simulink model "Pacemaker_Model"  (R2020a)
settings: Solver=FixedStepAuto  StartTime=0.0  StopTime=inf  FixedStep=1e-3  RelTol=1e-3  EnableMultiTasking=on
undefined symbols (not defined in the file): A0, A1, magnitude, PTB2, PTB3
libraries: etargetslib x7, frdmk64flib x5, dspstat3 x1
settings Model: ExtModeTrigDuration=5  Creator=iceca  LastModifiedBy=iceca
settings OptimizationCC: EnhancedBackFolding=on  PassReuseOutputArgsAs=Individual arguments  ZeroExternalMemoryAtStartup=off  ZeroInternalMemoryAtStartup=off  MaxStackSize=64  OptimizeBlockOrder=speed  DifferentSizesBufferReuse=on  OptimizationCustomize=off  EfficientTunableParamExpr=on
settings DebuggingCC: ParameterTunabilityLossMsg=error
settings HardwareCC: ProdBitPerPointer=32  ProdBitPerSizeT=32  ProdBitPerPtrDiffT=32  ProdLargestAtomicInteger=Long  ProdLargestAtomicFloat=Double  ProdWordSize=32  ProdHWDeviceType=ARM Compatible->ARM Cortex
settings SFSimCC: MATLABDynamicMemAlloc=off
settings RTWCC: SystemTargetFile=ert.tlc  HardwareBoard=NXP FRDM-K64F  TemplateMakefile=ert_default_tmf  Toolchain=GNU Tools for ARM Embedded Processors
settings CodeAppCC: ForceParamTrailComments=on  IgnoreCustomStorageClasses=off  OperatorAnnotations=on  SimulinkDataObjDesc=on  SFDataObjDesc=on  InsertBlockDesc=on

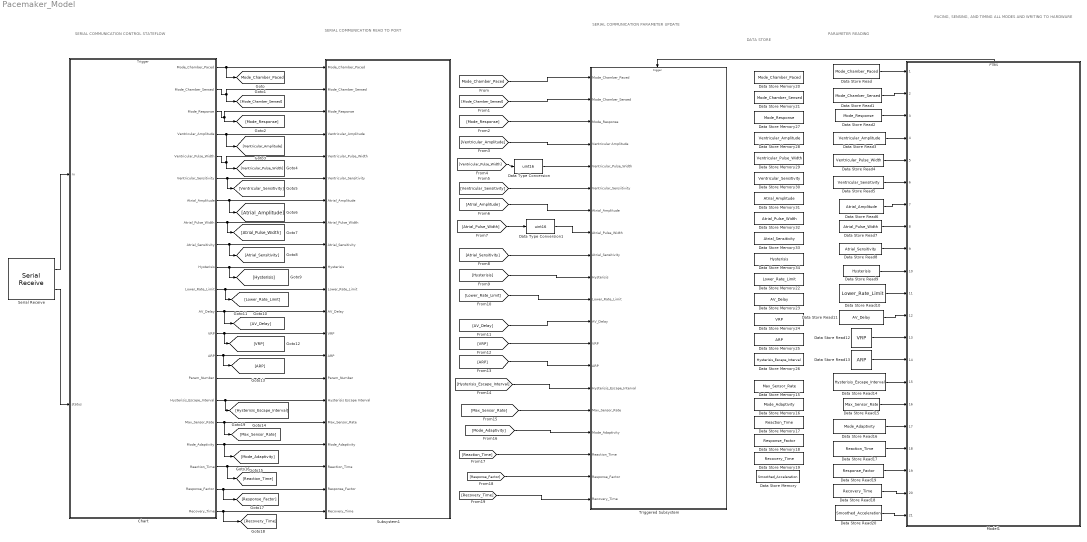
== system Pacemaker_Model ==
  note: SERIAL COMMUNICATION
      | CONTROL STATEFLOW
  note: SERIAL COMMUNICATION
      | READ TO PORT
  note: SERIAL COMMUNICATION
      | PARAMETER UPDATE
  note: DATA STORE
  note: PARAMETER
      | READING
  note: PACING, SENSING, AND TIMING
      | ALL MODES AND WRITING
      | TO HARDWARE
  Chart : Stateflow chart  TreatAsAtomicUnit=on
      settings: PortSchema="{\"entries\":[{\"content\":{\"sides\":[{\"content\":{\"connectorIds\":[\"In1\",\"In2\"]},\"type\":\"ConnectorPlacement.EquallySpacedRectSide\",\"uuid\":\"5d6148fe-63ad-4e41-a469-0ccea700ff5c\"},{\"content\":{\"connectorIds\":[\"Out2\",\"Out3\",\"Out4\",\"Out5\",\"Out6\",\"Out7\",\"Out8\",\"Out9\",\"Out10\",\"Out11\",\"Out12\",\"Out13\",\"Out14\",\"Out15\",\"Out17\",\"Out16\",\"Out18\",\"Out19\",\"Out20\",\"Out21\",\"Out22\"],\"side\":\"RIGHT\"},\"type\":\"ConnectorPlacement.EquallySpacedRectSide\",\"uuid\":\"22e91669-c20d-44ca-9338-cd13d2e9e618\"},{\"content\":{\"connectorIds\":[\"Out1\"],\"side\":\"TOP\"},\"type\":\"ConnectorPlacement.EquallySpacedRectSide\",\"uuid\":\"06f0f997-4aed-43a7-87af-d7ac7b59093d\"}]},\"type\":\"ConnectorPlacement.EquallySpacedConnector\",\"uuid\":\"618800eb-2d4f-49bb-a7f5-00e96badcb1e\"}],\"packageUris\":[\"http://schema.mathworks.com/mf0/Connector/19700101\"],\"version\":\"1.0\"}"
  Data Store Memory : DataStoreMemory  DataStoreName=Smoothed_Acceleration  ReadBeforeWriteMsg=warning  WriteAfterWriteMsg=warning  WriteAfterReadMsg=warning  ShowAdditionalParam=off
  Data Store Memory15 : DataStoreMemory  DataStoreName=Max_Sensor_Rate  ReadBeforeWriteMsg=warning  WriteAfterWriteMsg=warning  WriteAfterReadMsg=warning  ShowAdditionalParam=off
  Data Store Memory16 : DataStoreMemory  DataStoreName=Mode_Adaptivity  ReadBeforeWriteMsg=warning  WriteAfterWriteMsg=warning  WriteAfterReadMsg=warning  ShowAdditionalParam=off
  Data Store Memory17 : DataStoreMemory  DataStoreName=Reaction_Time  ReadBeforeWriteMsg=warning  WriteAfterWriteMsg=warning  WriteAfterReadMsg=warning  ShowAdditionalParam=off
  Data Store Memory18 : DataStoreMemory  DataStoreName=Response_Factor  ReadBeforeWriteMsg=warning  WriteAfterWriteMsg=warning  WriteAfterReadMsg=warning  ShowAdditionalParam=off
  Data Store Memory19 : DataStoreMemory  DataStoreName=Recovery_Time  ReadBeforeWriteMsg=warning  WriteAfterWriteMsg=warning  WriteAfterReadMsg=warning  ShowAdditionalParam=off
  Data Store Memory20 : DataStoreMemory  DataStoreName=Mode_Chamber_Paced  ReadBeforeWriteMsg=warning  WriteAfterWriteMsg=warning  WriteAfterReadMsg=warning  ShowAdditionalParam=off
  Data Store Memory21 : DataStoreMemory  DataStoreName=Mode_Chamber_Sensed  ReadBeforeWriteMsg=warning  WriteAfterWriteMsg=warning  WriteAfterReadMsg=warning  ShowAdditionalParam=off
  Data Store Memory22 : DataStoreMemory  DataStoreName=Lower_Rate_Limit  ReadBeforeWriteMsg=warning  WriteAfterWriteMsg=warning  WriteAfterReadMsg=warning  ShowAdditionalParam=off
  Data Store Memory23 : DataStoreMemory  DataStoreName=AV_Delay  ReadBeforeWriteMsg=warning  WriteAfterWriteMsg=warning  WriteAfterReadMsg=warning  ShowAdditionalParam=off
  Data Store Memory24 : DataStoreMemory  DataStoreName=VRP  ReadBeforeWriteMsg=warning  WriteAfterWriteMsg=warning  WriteAfterReadMsg=warning  ShowAdditionalParam=off
  Data Store Memory25 : DataStoreMemory  DataStoreName=ARP  ReadBeforeWriteMsg=warning  WriteAfterWriteMsg=warning  WriteAfterReadMsg=warning  ShowAdditionalParam=off
  Data Store Memory26 : DataStoreMemory  DataStoreName=Hysterisis_Escape_Interval  ReadBeforeWriteMsg=warning  WriteAfterWriteMsg=warning  WriteAfterReadMsg=warning  ShowAdditionalParam=off
  Data Store Memory27 : DataStoreMemory  DataStoreName=Mode_Response  ReadBeforeWriteMsg=warning  WriteAfterWriteMsg=warning  WriteAfterReadMsg=warning  ShowAdditionalParam=off
  Data Store Memory28 : DataStoreMemory  DataStoreName=Ventricular_Amplitude  ReadBeforeWriteMsg=warning  WriteAfterWriteMsg=warning  WriteAfterReadMsg=warning  ShowAdditionalParam=off
  Data Store Memory29 : DataStoreMemory  DataStoreName=Ventricular_Pulse_Width  ReadBeforeWriteMsg=warning  WriteAfterWriteMsg=warning  WriteAfterReadMsg=warning  ShowAdditionalParam=off
  Data Store Memory30 : DataStoreMemory  DataStoreName=Ventricular_Sensitivity  ReadBeforeWriteMsg=warning  WriteAfterWriteMsg=warning  WriteAfterReadMsg=warning  ShowAdditionalParam=off
  Data Store Memory31 : DataStoreMemory  DataStoreName=Atrial_Amplitude  ReadBeforeWriteMsg=warning  WriteAfterWriteMsg=warning  WriteAfterReadMsg=warning  ShowAdditionalParam=off
  Data Store Memory32 : DataStoreMemory  DataStoreName=Atrial_Pulse_Width  ReadBeforeWriteMsg=warning  WriteAfterWriteMsg=warning  WriteAfterReadMsg=warning  ShowAdditionalParam=off
  Data Store Memory33 : DataStoreMemory  DataStoreName=Atrial_Sensitivity  ReadBeforeWriteMsg=warning  WriteAfterWriteMsg=warning  WriteAfterReadMsg=warning  ShowAdditionalParam=off
  Data Store Memory34 : DataStoreMemory  DataStoreName=Hysterisis  ReadBeforeWriteMsg=warning  WriteAfterWriteMsg=warning  WriteAfterReadMsg=warning  ShowAdditionalParam=off
  Data Store Read : DataStoreRead  DataStoreName=Mode_Chamber_Paced
  Data Store Read1 : DataStoreRead  DataStoreName=Mode_Chamber_Sensed
  Data Store Read10 : DataStoreRead  DataStoreName=Lower_Rate_Limit
  Data Store Read11 : DataStoreRead  DataStoreName=AV_Delay
  Data Store Read12 : DataStoreRead  DataStoreName=VRP
  Data Store Read13 : DataStoreRead  DataStoreName=ARP
  Data Store Read14 : DataStoreRead  DataStoreName=Hysterisis_Escape_Interval
  Data Store Read15 : DataStoreRead  DataStoreName=Max_Sensor_Rate
  Data Store Read16 : DataStoreRead  DataStoreName=Mode_Adaptivity
  Data Store Read17 : DataStoreRead  DataStoreName=Reaction_Time
  Data Store Read18 : DataStoreRead  DataStoreName=Recovery_Time
  Data Store Read19 : DataStoreRead  DataStoreName=Response_Factor
  Data Store Read2 : DataStoreRead  DataStoreName=Mode_Response
  Data Store Read20 : DataStoreRead  DataStoreName=Smoothed_Acceleration
  Data Store Read3 : DataStoreRead  DataStoreName=Ventricular_Amplitude
  Data Store Read4 : DataStoreRead  DataStoreName=Ventricular_Pulse_Width
  Data Store Read5 : DataStoreRead  DataStoreName=Ventricular_Sensitivity
  Data Store Read6 : DataStoreRead  DataStoreName=Atrial_Amplitude
  Data Store Read7 : DataStoreRead  DataStoreName=Atrial_Pulse_Width
  Data Store Read8 : DataStoreRead  DataStoreName=Atrial_Sensitivity
  Data Store Read9 : DataStoreRead  DataStoreName=Hysterisis
  Data Type Conversion : DataTypeConversion  OutDataTypeStr=uint16
  Data Type Conversion1 : DataTypeConversion  OutDataTypeStr=uint16
  Model1 : ModelReference  ModelNameDialog=PTHS.slx  SimulationMode=Normal  ModelReferenceVersion=1.35
      settings: PortSchema="{\"entries\":[{\"content\":{\"sides\":[{\"content\":{\"connectorIds\":[\"In1\",\"In2\",\"In3\",\"In4\",\"In5\",\"In6\",\"In7\",\"In8\",\"In9\",\"In10\",\"In11\",\"In12\",\"In13\",\"In14\",\"In15\",\"In16\",\"In17\",\"In18\",\"In19\",\"In20\",\"In21\"]},\"type\":\"ConnectorPlacement.EquallySpacedRectSide\",\"uuid\":\"589ed8b8-76bd-4f54-af86-3c44c90fe378\"},{\"content\":{\"connectorIds\":[],\"side\":\"RIGHT\"},\"type\":\"ConnectorPlacement.EquallySpacedRectSide\",\"uuid\":\"907c2eb9-05aa-466e-8747-34035dc70ead\"},{\"content\":{\"connectorIds\":[\"Out1\"],\"side\":\"TOP\"},\"type\":\"ConnectorPlacement.EquallySpacedRectSide\",\"uuid\":\"d1beb45c-33da-41d8-bf39-7e12395cad16\"}]},\"type\":\"ConnectorPlacement.EquallySpacedConnector\",\"uuid\":\"0af1fbfe-4207-406c-aebc-86d3337d36f5\"}],\"packageUris\":[\"http://schema.mathworks.com/mf0/Connector/19700101\"],\"version\":\"1.0\"}"
  Serial Receive : frdmk64flib/Serial Receive  SCIModule=0  Baudrate=uint32(9600)  Parity=None  StopBits=1  HardwareFlowControl=None  ByteOrder=LittleEndian  DataType=uint8  DataLength=27  BlockingMode=off  OutputStatus=on  SampleTime=-1
  Subsystem1 : Subsystem
  Triggered Subsystem : Subsystem  TreatAsAtomicUnit=on
  tag scope: Mode_Chamber_Paced=global
  wires:
  Serial Receive/1 -> Chart/1(rx)
  Serial Receive/2 -> Chart/2(status)
  Chart/2(Mode_Chamber_Paced) -> Subsystem1/1(Mode_Chamber_Paced), [Mode_Chamber_Paced]
  Chart/11(Hysterisis) -> [Hysterisis], Subsystem1/10(Hysterisis)
  Chart/12(Lower_Rate_Limit) -> [Lower_Rate_Limit], Subsystem1/11(Lower_Rate_Limit)
  Chart/13(AV_Delay) -> [AV_Delay], Subsystem1/12(AV_Delay)
  Chart/14(VRP) -> [VRP], Subsystem1/13(VRP)
  Chart/15(ARP) -> [ARP], Subsystem1/14(ARP)
  Chart/16(Hysterisis_Escape_Interval) -> [Hysterisis_Escape_Interval], Subsystem1/16(Hysterisis Escape Interval)
  Chart/3(Mode_Chamber_Sensed) -> Subsystem1/2(Mode_Chamber_Sensed), [Mode_Chamber_Sensed]
  Chart/4(Mode_Response) -> Subsystem1/3(Mode_Response), [Mode_Response]
  Chart/5(Ventricular_Amplitude) -> Subsystem1/4(Ventricular_Amplitude), [Ventricular_Amplitude]
  Chart/7(Ventricular_Sensitivity) -> [Ventricular_Sensitivity], Subsystem1/6(Ventricular_Sensitivity)
  Chart/8(Atrial_Amplitude) -> [Atrial_Amplitude], Subsystem1/7(Atrial_Amplitude)
  Chart/10(Atrial_Sensitivity) -> [Atrial_Sensitivity], Subsystem1/9(Atrial_Sensitivity)
  Chart/6(Ventricular_Pulse_Width) -> Subsystem1/5(Ventricular_Pulse_Width), [Ventricular_Pulse_Width]
  Chart/9(Atrial_Pulse_Width) -> [Atrial_Pulse_Width], Subsystem1/8(Atrial_Pulse_Width)
  [Ventricular_Pulse_Width] -> Data Type Conversion/1
  [Atrial_Pulse_Width] -> Data Type Conversion1/1
  Chart/18(Max_Sensor_Rate) -> [Max_Sensor_Rate], Subsystem1/17(Max_Sensor_Rate)
  Chart/19(Mode_Adaptivity) -> Subsystem1/18(Mode_Adaptivity), [Mode_Adaptivity]
  Chart/17(Param_Number) -> Subsystem1/15(Param_Number)
  Chart/22(Recovery_Time) -> Subsystem1/21(Recovery_Time), [Recovery_Time]
  Chart/20(Reaction_Time) -> [Reaction_Time], Subsystem1/19(Reaction_Time)
  Chart/21(Response_Factor) -> [Response_Factor], Subsystem1/20(Response_Factor)
  [Mode_Chamber_Paced] -> Triggered Subsystem/1(Mode_Chamber_Paced)
  [Mode_Chamber_Sensed] -> Triggered Subsystem/2(Mode_Chamber_Sensed)
  [Ventricular_Amplitude] -> Triggered Subsystem/4(Ventricular Amplitude)
  [Mode_Response] -> Triggered Subsystem/3(Mode_Response)
  [Ventricular_Sensitivity] -> Triggered Subsystem/6(Ventricular_Sensiitivity)
  Data Type Conversion/1 -> Triggered Subsystem/5(Ventricular_Pulse_Width)
  [Atrial_Amplitude] -> Triggered Subsystem/7(Atrial_Amplitude)
  Data Type Conversion1/1 -> Triggered Subsystem/8(Atrial_Pulse_Width)
  [Atrial_Sensitivity] -> Triggered Subsystem/9(Atrial_Sensitivity)
  [Hysterisis] -> Triggered Subsystem/10(Hysterisis)
  [AV_Delay] -> Triggered Subsystem/12(AV_Delay)
  [VRP] -> Triggered Subsystem/13(VRP)
  [ARP] -> Triggered Subsystem/14(ARP)
  [Hysterisis_Escape_Interval] -> Triggered Subsystem/15(Hysterisis_Escape_Interval)
  [Mode_Adaptivity] -> Triggered Subsystem/17(Mode_Adaptivity)
  [Reaction_Time] -> Triggered Subsystem/18(Reaction_Time)
  [Response_Factor] -> Triggered Subsystem/19(Response_Factor)
  [Recovery_Time] -> Triggered Subsystem/20(Recovery_Time)
  Model1/1 -> Triggered Subsystem/Trigger
  [Max_Sensor_Rate] -> Triggered Subsystem/16(Max_Sensor_Rate)
  Data Store Read/1 -> Model1/1
  Data Store Read1/1 -> Model1/2
  Data Store Read2/1 -> Model1/3
  Data Store Read3/1 -> Model1/4
  Data Store Read4/1 -> Model1/5
  Data Store Read5/1 -> Model1/6
  Data Store Read6/1 -> Model1/7
  Data Store Read7/1 -> Model1/8
  Data Store Read8/1 -> Model1/9
  Data Store Read9/1 -> Model1/10
  Data Store Read10/1 -> Model1/11
  Data Store Read11/1 -> Model1/12
  Data Store Read12/1 -> Model1/13
  Data Store Read13/1 -> Model1/14
  Data Store Read14/1 -> Model1/15
  [Lower_Rate_Limit] -> Triggered Subsystem/11(Lower_Rate_Limit)
  Data Store Read15/1 -> Model1/16
  Data Store Read16/1 -> Model1/17
  Data Store Read17/1 -> Model1/18
  Data Store Read18/1 -> Model1/20
  Data Store Read19/1 -> Model1/19
  Data Store Read20/1 -> Model1/21

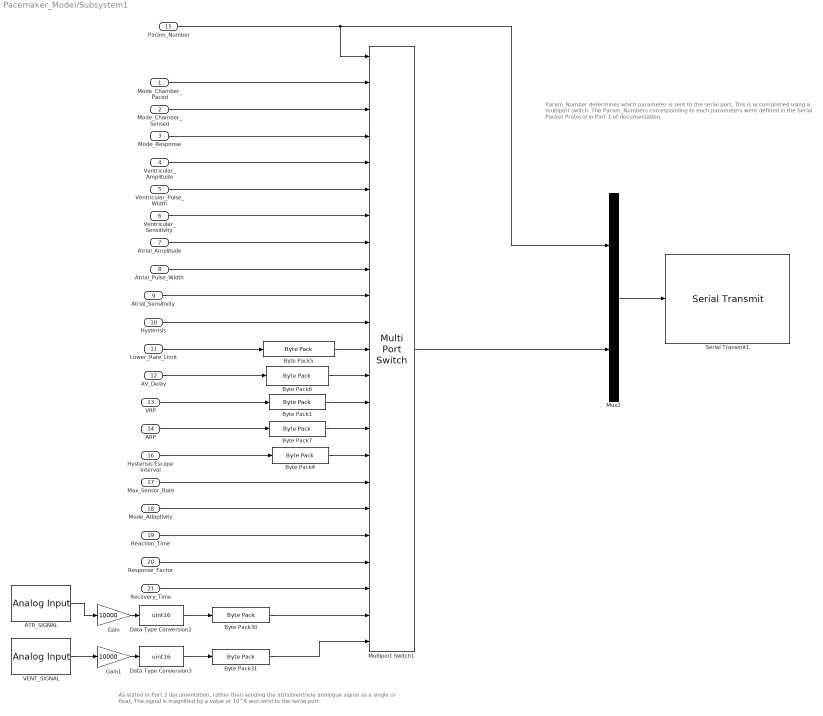
== system Pacemaker_Model/Subsystem1 ==
  note: As stated in Part 2 documentation, rather then sending the atrial/ventricle analogue signal as a single or float,
      | The signal is magnified by a value of 10^4 and send to the serial port.
  note: Param_Number determines which parameter is sent to the serial port.
      | This is accomplished using a multiport switch.
      | The Param_Numbers corresponding to each parameters were defined in the
      | Serial Packet Protocol in Part 1 of documentation.
  Mode_Chamber_Paced : Inport
  Mode_Chamber_Sensed : Inport  Port=2
  Mode_Response : Inport  Port=3
  Ventricular_Amplitude : Inport  Port=4
  Ventricular_Pulse_Width : Inport  Port=5
  Ventricular_Sensitivity : Inport  Port=6
  Atrial_Amplitude : Inport  Port=7
  Atrial_Pulse_Width : Inport  Port=8
  Atrial_Sensitivity : Inport  Port=9
  Hysterisis : Inport  Port=10
  Lower_Rate_Limit : Inport  Port=11
  AV_Delay : Inport  Port=12
  VRP : Inport  Port=13
  ARP : Inport  Port=14
  Param_Number : Inport  Port=15
  Hysterisis Escape Interval : Inport  Port=16
  Max_Sensor_Rate : Inport  Port=17
  Mode_Adaptivity : Inport  Port=18
  Reaction_Time : Inport  Port=19
  Response_Factor : Inport  Port=20
  Recovery_Time : Inport  Port=21
  ATR_SIGNAL : frdmk64flib/Analog Input  Whichpin=PTB2 (A0)  SampleTime=-1
  Byte Pack{1,4..7,30..31} (7 alike) : etargetslib/Byte Pack  datatypes={'uint16'}  byteAlign=1
  Data Type Conversion2 : DataTypeConversion  OutDataTypeStr=uint16
  Data Type Conversion3 : DataTypeConversion  OutDataTypeStr=uint16
  Gain : Gain  Gain=10000
  Gain1 : Gain  Gain=10000
  Multiport Switch1 : MultiPortSwitch  Inputs=22
  Mux2 : Mux  Inputs=2
  Serial Transmit1 : frdmk64flib/Serial Transmit  SCIModule=0  Baudrate=uint32(9600)  Parity=None  StopBits=1  HardwareFlowControl=None  ByteOrder=LittleEndian  BlockingMode=on  OutputStatus=off
  VENT_SIGNAL : frdmk64flib/Analog Input  Whichpin=PTB3 (A1)  SampleTime=-1
  wires:
  Lower_Rate_Limit/1 -> Byte Pack5/1
  ARP/1 -> Byte Pack7/1
  VRP/1 -> Byte Pack1/1
  Hysterisis Escape Interval/1 -> Byte Pack4/1
  AV_Delay/1 -> Byte Pack6/1
  Param_Number/1 -> Mux2/1, Multiport Switch1/1
  Mode_Response/1 -> Multiport Switch1/4
  Mode_Chamber_Sensed/1 -> Multiport Switch1/3
  Mode_Chamber_Paced/1 -> Multiport Switch1/2
  Ventricular_Amplitude/1 -> Multiport Switch1/5
  Ventricular_Pulse_Width/1 -> Multiport Switch1/6
  Ventricular_Sensitivity/1 -> Multiport Switch1/7
  Atrial_Amplitude/1 -> Multiport Switch1/8
  Atrial_Pulse_Width/1 -> Multiport Switch1/9
  Atrial_Sensitivity/1 -> Multiport Switch1/10
  Hysterisis/1 -> Multiport Switch1/11
  Byte Pack5/1 -> Multiport Switch1/12
  Byte Pack6/1 -> Multiport Switch1/13
  Byte Pack1/1 -> Multiport Switch1/14
  Byte Pack7/1 -> Multiport Switch1/15
  Byte Pack4/1 -> Multiport Switch1/16
  Max_Sensor_Rate/1 -> Multiport Switch1/17
  Mode_Adaptivity/1 -> Multiport Switch1/18
  Reaction_Time/1 -> Multiport Switch1/19
  Response_Factor/1 -> Multiport Switch1/20
  Recovery_Time/1 -> Multiport Switch1/21
  Multiport Switch1/1 -> Mux2/2
  Mux2/1 -> Serial Transmit1/1
  ATR_SIGNAL/1 -> Gain/1
  Gain/1 -> Data Type Conversion2/1
  Data Type Conversion2/1 -> Byte Pack30/1
  Byte Pack30/1 -> Multiport Switch1/22
  Gain1/1 -> Data Type Conversion3/1
  Data Type Conversion3/1 -> Byte Pack31/1
  VENT_SIGNAL/1 -> Gain1/1
  Byte Pack31/1 -> Multiport Switch1/23

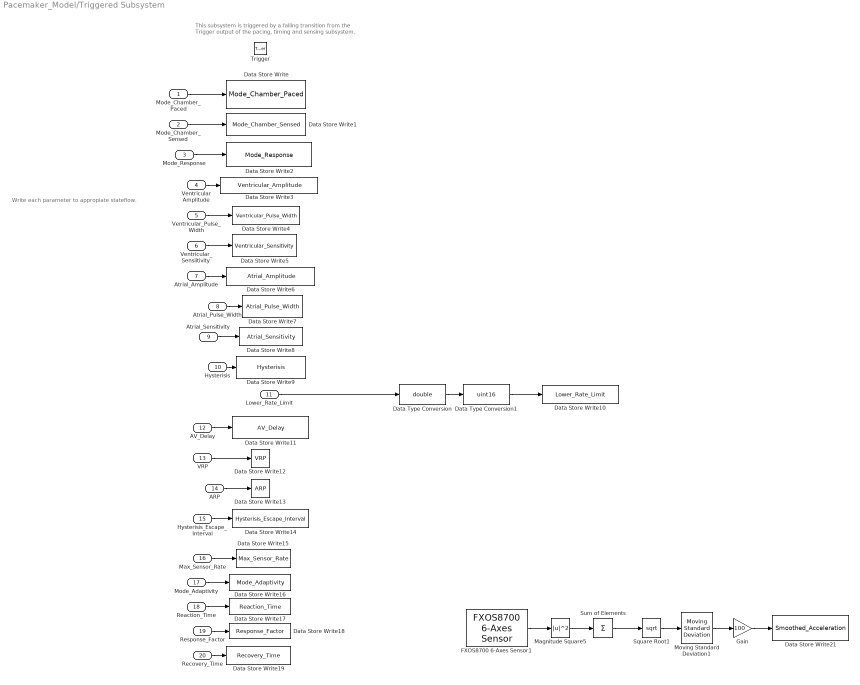
== system Pacemaker_Model/Triggered Subsystem ==
  note: This subsystem is triggered by a falling transition from the
      | Trigger output of the pacing, timing and sensing subsystem.
  note: Write each parameter to appropiate stateflow.
  Mode_Chamber_Paced : Inport
  Mode_Chamber_Sensed : Inport  Port=2
  Mode_Response : Inport  Port=3
  Ventricular Amplitude : Inport  Port=4
  Ventricular_Pulse_Width : Inport  Port=5
  Ventricular_Sensiitivity : Inport  Port=6
  Atrial_Amplitude : Inport  Port=7
  Atrial_Pulse_Width : Inport  Port=8
  Atrial_Sensitivity : Inport  Port=9
  Hysterisis : Inport  Port=10
  Lower_Rate_Limit : Inport  Port=11
  AV_Delay : Inport  Port=12
  VRP : Inport  Port=13
  ARP : Inport  Port=14
  Hysterisis_Escape_Interval : Inport  Port=15
  Max_Sensor_Rate : Inport  Port=16
  Mode_Adaptivity : Inport  Port=17
  Reaction_Time : Inport  Port=18
  Response_Factor : Inport  Port=19
  Recovery_Time : Inport  Port=20
  Trigger : TriggerPort  TriggerType=falling  VariantControl=Variant
  Data Store Write : DataStoreWrite  DataStoreName=Mode_Chamber_Paced
  Data Store Write1 : DataStoreWrite  DataStoreName=Mode_Chamber_Sensed
  Data Store Write10 : DataStoreWrite  DataStoreName=Lower_Rate_Limit
  Data Store Write11 : DataStoreWrite  DataStoreName=AV_Delay
  Data Store Write12 : DataStoreWrite  DataStoreName=VRP
  Data Store Write13 : DataStoreWrite  DataStoreName=ARP
  Data Store Write14 : DataStoreWrite  DataStoreName=Hysterisis_Escape_Interval
  Data Store Write15 : DataStoreWrite  DataStoreName=Max_Sensor_Rate
  Data Store Write16 : DataStoreWrite  DataStoreName=Mode_Adaptivity
  Data Store Write17 : DataStoreWrite  DataStoreName=Reaction_Time
  Data Store Write18 : DataStoreWrite  DataStoreName=Response_Factor
  Data Store Write19 : DataStoreWrite  DataStoreName=Recovery_Time
  Data Store Write2 : DataStoreWrite  DataStoreName=Mode_Response
  Data Store Write21 : DataStoreWrite  DataStoreName=Smoothed_Acceleration
  Data Store Write3 : DataStoreWrite  DataStoreName=Ventricular_Amplitude
  Data Store Write4 : DataStoreWrite  DataStoreName=Ventricular_Pulse_Width
  Data Store Write5 : DataStoreWrite  DataStoreName=Ventricular_Sensitivity
  Data Store Write6 : DataStoreWrite  DataStoreName=Atrial_Amplitude
  Data Store Write7 : DataStoreWrite  DataStoreName=Atrial_Pulse_Width
  Data Store Write8 : DataStoreWrite  DataStoreName=Atrial_Sensitivity
  Data Store Write9 : DataStoreWrite  DataStoreName=Hysterisis
  Data Type Conversion : DataTypeConversion  OutDataTypeStr=double
  Data Type Conversion1 : DataTypeConversion  OutDataTypeStr=uint16
  FXOS8700 6-Axes Sensor1 : frdmk64flib/FXOS8700 6-Axes Sensor  Activesensor=Accelerometer only  ODR=800Hz  HybridODR=400Hz  Accelfullrange=-2g to +2g  SampleTime=-1
  Gain : Gain  Gain=100
  Magnitude Square5 : Math  Operator=magnitude^2  SignedPower=on  RndMeth=Zero  SaturateOnIntegerOverflow=on
  Moving Standard Deviation1 : dspstat3/Moving Standard Deviation  Method=Sliding window  ForgettingFactorPort=off  SpecifyWindowLength=on  WindowLength=3  ForgettingFactor=0.9  SimulateUsing=Code generation
      settings: SourceProductBaseCode=DS
  Square Root1 : Sqrt  SaturateOnIntegerOverflow=on
  Sum of Elements : Sum  Inputs=+
  wires:
  Mode_Chamber_Paced/1 -> Data Store Write/1
  Mode_Chamber_Sensed/1 -> Data Store Write1/1
  Mode_Response/1 -> Data Store Write2/1
  Ventricular Amplitude/1 -> Data Store Write3/1
  Ventricular_Pulse_Width/1 -> Data Store Write4/1
  Ventricular_Sensiitivity/1 -> Data Store Write5/1
  Atrial_Amplitude/1 -> Data Store Write6/1
  Atrial_Pulse_Width/1 -> Data Store Write7/1
  VRP/1 -> Data Store Write12/1
  Atrial_Sensitivity/1 -> Data Store Write8/1
  Hysterisis/1 -> Data Store Write9/1
  ARP/1 -> Data Store Write13/1
  AV_Delay/1 -> Data Store Write11/1
  Hysterisis_Escape_Interval/1 -> Data Store Write14/1
  Mode_Adaptivity/1 -> Data Store Write16/1
  Reaction_Time/1 -> Data Store Write17/1
  Response_Factor/1 -> Data Store Write18/1
  Recovery_Time/1 -> Data Store Write19/1
  Max_Sensor_Rate/1 -> Data Store Write15/1
  Lower_Rate_Limit/1 -> Data Type Conversion/1
  Data Type Conversion/1 -> Data Type Conversion1/1
  Data Type Conversion1/1 -> Data Store Write10/1
  Square Root1/1 -> Moving Standard Deviation1/1
  FXOS8700 6-Axes Sensor1/1 -> Magnitude Square5/1
  Magnitude Square5/1 -> Sum of Elements/1
  Sum of Elements/1 -> Square Root1/1
  Moving Standard Deviation1/1 -> Gain/1
  Gain/1 -> Data Store Write21/1

== stateflow chart Pacemaker_Model/Chart ==
  state WRITE_PARAMS
    entry:
    %See Serial Protocol section in Part 1 of documentation
    %OFFSET
    %A local variable offset is used to index rx instead of raw numbers
    offset=3;
    %MODES
    Mode_Chamber_Paced=rx(offset);
    offset=offset+uint8_bytes;
    Mode_Chamber_Sensed=rx(offset);
    offset=offset+uint8_bytes;
    Mode_Response=rx(offset);
    offset=offset+uint8_bytes;
    %VENTRICLULAR PACE PARAMS
    Ventricular_Amplitude=rx(offset);
    offset=offset+uint8_bytes;
    Ventricular_Pulse_Width=rx(offset);
    offset=offset+uint8_bytes;
    Ventricular_Sensitivity=rx(offset);
    offset=offset+uint8_bytes;
    %ATRIAL PACE PARAMS
    Atrial_Amplitude=rx(offset);
    offset=offset+uint8_bytes;
    Atrial_Pulse_Width=rx(offset);
    offset=offset+uint8_bytes;
    Atrial_Sensitivity=rx(offset);
    offset=offset+uint8_bytes;
    %HYSTERISIS
    Hysterisis=rx(offset);
    offset=offset+uint8_bytes;
    %uint16 PARAMETERS
    Lower_Rate_Limit=typecast(rx(offset:offset+1),'uint16');
    offset=offset+uint16_bytes;
    AV_Delay=typecast(rx(offset:offset+1),'uint16');
    offset=offset+uint16_bytes;
    VRP=typecast(rx(offset:offset+1),'uint16');
    offset=offset+uint16_bytes;
    ARP=typecast(rx(offset:offset+1),'uint16');
    offset=offset+uint16_bytes;
    Hysterisis_Escape_Interval=typecast(rx(offset:offset+1),'uint16');
    offset=offset+uint16_bytes;
    %RATE ADAPTIVITY
    Max_Sensor_Rate = rx(offset);
    offset=offset+uint8_bytes;
    Mode_Adaptivity = rx(offset);
    offset=offset+uint8_bytes;
    Reaction_Time=rx(offset);
    offset=offset+uint8_bytes;
    Response_Factor = rx(offset);
    offset=offset+uint8_bytes;
    Recovery_Time =  rx(offset);
    offset=offset+uint8_bytes;
  note: TEST_CODE: 10
      | SET_CODE: 20
      | ECHO_CODE: 30
  state START_STATE
    entry:
    uint16_bytes = 2;
    uint8_bytes = 1;
    single_bytes=4;
  state WAIT_STATE
    entry:
    Trigger = false;
  state READ_PARAMS
    entry:
    %See Serial Protocol section in Part 1 of documentation
    Param_Number=rx(3);
    Trigger = true;
  WRITE_PARAMS -> WAIT_STATE
  (junction 199) -> WRITE_PARAMS [order 1] : [rx(2)==20]
  (default) -> START_STATE
  (junction 132) -> WAIT_STATE [order 2]
  START_STATE -> WAIT_STATE
  WAIT_STATE -> (junction 132) : [status == 0]
  (junction 132) -> (junction 199) [order 1] : [rx(1)==10]
  (junction 199) -> READ_PARAMS [order 2] : [rx(2) == 30]
  READ_PARAMS -> WAIT_STATE
  data: Trigger output; Mode_Chamber_Paced output; Mode_Chamber_Sensed output; Mode_Response output; Ventricular_Amplitude output; Ventricular_Pulse_Width output; Ventricular_Sensitivity output; Atrial_Amplitude output; rx input uint8; offset local; Atrial_Pulse_Width output; Atrial_Sensitivity output; Hysterisis output; Lower_Rate_Limit output; AV_Delay output; VRP output; ARP output; Hysterisis_Escape_Interval output; status input uint8; uint16_bytes local; uint8_bytes local; single_bytes local; Param_Number output; Max_Sensor_Rate output; Mode_Adaptivity output; Reaction_Time output; Response_Factor output; Recovery_Time output
